simulink model "rocky"  (R2023b)
settings: Solver=VariableStepAuto  StartTime=0.0  StopTime=10.0  RelTol=1e-3
values from neighbouring files (symbols this model uses):
  a = (1/0.0661+1/0.0659)/2    (= 15.1515499347)    [Rocky_5_closed_loop_poles.m]    (also in Rocky_closed_loop_poles_24.m)
  b = (0.0028+0.0030)/2    (= 0.0029)    [Rocky_5_closed_loop_poles.m]    (also in Rocky_closed_loop_poles_24.m)
  Ci = real(double(solutions.Ci))    [Rocky_5_closed_loop_poles.m]
  g = 9.81    [Rocky_5_closed_loop_poles.m]    (also in Rocky_closed_loop_poles_24.m)
  Ji = real(double(solutions.Ji))    [Rocky_5_closed_loop_poles.m]
  Jp = real(double(solutions.Jp))    [Rocky_5_closed_loop_poles.m]
  Ki = real(double(solutions.Ki))    [Rocky_5_closed_loop_poles.m]    (also in Rocky_closed_loop_poles_24.m = double(solutions.Ki))
  Kp = real(double(solutions.Kp))    [Rocky_5_closed_loop_poles.m]    (also in Rocky_closed_loop_poles_24.m = double(solutions.Kp))
  l = 0.4529    [Rocky_5_closed_loop_poles.m]    (also in Rocky_closed_loop_poles_24.m)
settings Model: Creator=liloa  LastModifiedBy=liloa

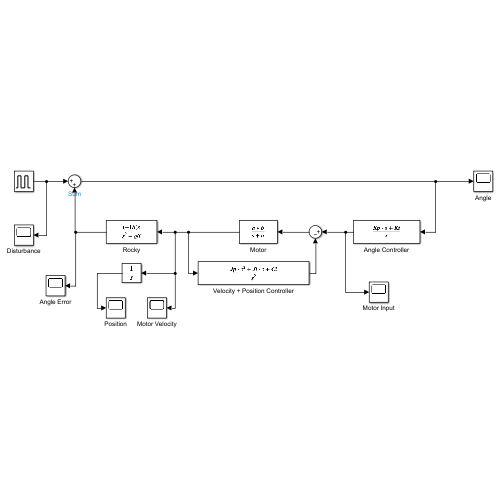
[thumbnail: Simulink's stored preview of the top-level diagram]
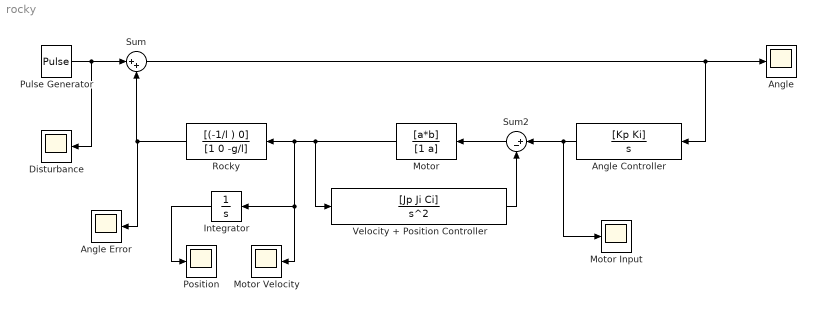
== system rocky ==
  Angle : Scope
  Angle Controller : TransferFcn  Numerator=[Kp Ki]  Denominator=[1 0]  ContinuousStateAttributes="\"MotorControl\""
  Angle Error : Scope
  Disturbance : Scope
  Integrator : Integrator
  Motor : TransferFcn  Numerator=[a*b]  Denominator=[1 a]  ContinuousStateAttributes="\"Motor\""
  Motor Input : Scope
  Motor Velocity : Scope
  Position : Scope
  Pulse Generator : DiscretePulseGenerator  PulseType=Time based  Period=60  PulseWidth=5
  Rocky : TransferFcn  Numerator=[(-1/l ) 0]  Denominator=[1 0 -g/l]  ContinuousStateAttributes="\"Rocky\""
  Sum : Sum  Inputs=|++
  Sum2 : Sum  Inputs=|+-
  Velocity + Position Controller : TransferFcn  Numerator=[Jp Ji Ci]  Denominator=[1 0 0]  ContinuousStateAttributes="\"VelocityControl\""
  wires:
  Pulse Generator/1 -> Disturbance/1, Sum/1
  Sum/1 -> Angle Controller/1, Angle/1
  Angle Controller/1 -> Sum2/1, Motor Input/1
  Rocky/1 -> Angle Error/1, Sum/2
  Integrator/1 -> Position/1
  Motor/1 -> Velocity + Position Controller/1, Motor Velocity/1, Integrator/1, Rocky/1
  Sum2/1 -> Motor/1
  Velocity + Position Controller/1 -> Sum2/2
